simulink model "IMUnav"  (R2017b)
settings: Solver=VariableStepAuto  StartTime=0.0  StopTime=inf  RelTol=1e-3
InitFcn:
  | init
undefined symbols (not defined in the file or in its folder): CR, LF, none, serial, videoinput
libraries: imaqlib x2, instrumentlib x2
settings Model: Creator=KingBoy  LastModifiedBy=KingBoy

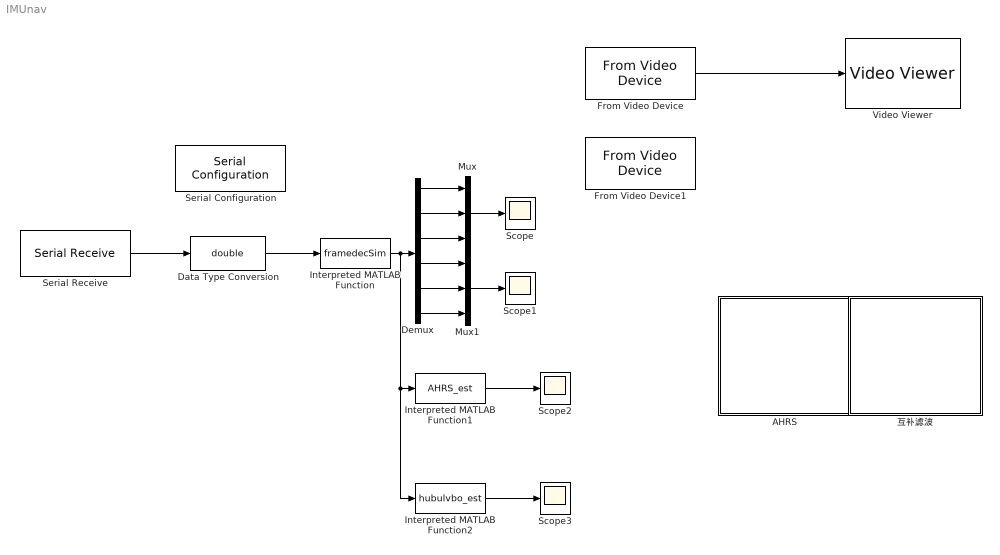
== system IMUnav ==
  AHRS : Subsystem  DialogController=aeroblksHMICreateDDGDialog  IsWebBlock=on  mask(MWDashboardBlock){webBlockId=c40ec512-5aa2-4241-a4b5-422d4a4aa7f9, webBlockType=artificialhorizon, ShowInLibBrowser=on, ShowInitialText=on, HMISrcModelName=IMUnav}
      mask prompts: webBlockId "WebBlock Id"; webBlockType "WebBlock Type"; HMISrcModelName "Source Model"
      mask help: aeroblksHMI:aeroblkhmi:ArtificialHorizonDialogDesc
      mask Help: eval('asbhmihelp(''artificialhorizon'')');
      mask Display:
      | if strcmp(get_param(bdroot(gcb),'BlockDiagramType'), 'library')
      |  image([(matlabroot) '/toolbox/aeroblks/aeroblks/hmi/icons/ArtificialHorizonIcon.svg'])
      | end
  Data Type Conversion : DataTypeConversion  OutDataTypeStr=double
  Demux : Demux  Outputs=6
  From Video Device : imaqlib/From Video Device  DeviceMenu=winvideo 1 (USB2.0 PC CAMERA)  Device=winvideo 1 (USB2.0 PC CAMERA)  ObjConstructor=videoinput('winvideo', 1)  VideoFormatMenu=YUY2_320x240  VideoFormat=YUY2_320x240  VideoSource=input1  ROIPosition=[0 0 240 320]  EnableHWTrigger=off  TriggerConfiguration=none/none  SampleTime=1/60  OutputPortsMode=One multidimensional signal  DataType=uint8  CanDoHWTrigger=no  ReturnedColorSpace=grayscale  BlockHandle=1831.0002  ROIWidth=320  ROIHeight=240  ROIColumn=0  ROIRow=0  EngXMLPath=C:\Program Files\MATLAB\R2017b\toolbox\imaq\imaq\private  DevXMLPath=C:\ProgramData\MATLAB\SupportPackages\R2017b\toolbox\imaq\supportpackages\genericvideo\adaptor\win64  EngLibPath=C:\Program Files\MATLAB\R2017b\toolbox\imaq\imaqblks\imaqmex\win64  ColorSpace=grayscale  BayerSensorAlignment=grbg
      settings: SourceProductName=Image Acquisition Toolbox
  From Video Device1 : imaqlib/From Video Device  DeviceMenu=winvideo 1 (USB2.0 PC CAMERA)  Device=winvideo 1 (USB2.0 PC CAMERA)  ObjConstructor=videoinput('winvideo', 1)  VideoFormatMenu=YUY2_320x240  VideoFormat=YUY2_320x240  VideoSource=input1  ROIPosition=[0 0 240 320]  EnableHWTrigger=off  TriggerConfiguration=none/none  SampleTime=1/60  OutputPortsMode=One multidimensional signal  DataType=uint8  CanDoHWTrigger=no  ReturnedColorSpace=grayscale  BlockHandle=1831.0002  ROIWidth=320  ROIHeight=240  ROIColumn=0  ROIRow=0  EngXMLPath=C:\Program Files\MATLAB\R2017b\toolbox\imaq\imaq\private  DevXMLPath=C:\ProgramData\MATLAB\SupportPackages\R2017b\toolbox\imaq\supportpackages\genericvideo\adaptor\win64  EngLibPath=C:\Program Files\MATLAB\R2017b\toolbox\imaq\imaqblks\imaqmex\win64  ColorSpace=grayscale  BayerSensorAlignment=grbg
      settings: SourceProductName=Image Acquisition Toolbox
  Interpreted MATLAB Function : MATLABFcn  MATLABFcn=framedecSim  OutputDimensions=6
  Interpreted MATLAB Function1 : MATLABFcn  MATLABFcn=AHRS_est  OutputDimensions=2
  Interpreted MATLAB Function2 : MATLABFcn  MATLABFcn=hubulvbo_est  OutputDimensions=2
  Mux : Mux  Inputs=3
  Mux1 : Mux  Inputs=3
  Scope{,1..3} (4 alike) : Scope
  Serial Configuration : instrumentlib/Serial Configuration  Priority=-200000  ComPortMenu=<Please select a port...>  ComPort=COM3  ObjConstructor=serial('COM3');  BaudRate=9600  DataBits=8  Parity=none  StopBits=1  FlowControl=none  Timeout=10  ByteOrder=LittleEndian
  Serial Receive : instrumentlib/Serial Receive  ComPortMenu=<Please select a port...>  ComPort=COM3  ObjConstructor=serial('COM3');  Header=$  Terminator=CR/LF ('\r\n')  DataSize="[27   1]"  DataType=uint8  EnableBlockingMode=on  ActionDataUnavailable=Output last received value  CustomValue=0  SampleTime=0.01
  Video Viewer : VideoViewer  FigPos=[1013 704 418 304]
  互补滤波 : Subsystem  DialogController=aeroblksHMICreateDDGDialog  IsWebBlock=on  mask(MWDashboardBlock){webBlockId=e0c47791-5582-4f28-97c7-f80d8fa19122, webBlockType=artificialhorizon, ShowInLibBrowser=on, ShowInitialText=on, HMISrcModelName=IMUnav}
      mask prompts: webBlockId "WebBlock Id"; webBlockType "WebBlock Type"; HMISrcModelName "Source Model"
      mask help: aeroblksHMI:aeroblkhmi:ArtificialHorizonDialogDesc
      mask Help: eval('asbhmihelp(''artificialhorizon'')');
      mask Display:
      | if strcmp(get_param(bdroot(gcb),'BlockDiagramType'), 'library')
      |  image([(matlabroot) '/toolbox/aeroblks/aeroblks/hmi/icons/ArtificialHorizonIcon.svg'])
      | end
  wires:
  Serial Receive/1 -> Data Type Conversion/1
  Interpreted MATLAB Function/1 -> Interpreted MATLAB Function2/1, Interpreted MATLAB Function1/1, Demux/1
  Demux/1 -> Mux/1
  Demux/2 -> Mux/2
  Demux/3 -> Mux/3
  Demux/4 -> Mux1/1
  Demux/5 -> Mux1/2
  Demux/6 -> Mux1/3
  Mux/1 -> Scope/1
  Mux1/1 -> Scope1/1
  Data Type Conversion/1 -> Interpreted MATLAB Function/1
  Interpreted MATLAB Function1/1 -> Scope2/1
  Interpreted MATLAB Function2/1 -> Scope3/1
  From Video Device/1 -> Video Viewer/1

== system IMUnav/AHRS ==

== system IMUnav/互补滤波 ==
